simulink model "TP3_simu_realim_obs_continuo"  (R2023b)
settings: Solver=VariableStepAuto  StartTime=0.0  StopTime=6  FixedStep=20e-3  RelTol=1e-3
values from neighbouring files (symbols this model uses):
  A = sysc .A    [Prueba_Control.m]
  B = sysc .B    [Prueba_Control.m]
  C = sysc .C    [Prueba_Control.m]
  D = sysc .D    [Prueba_Control.m]
  x1e = 0    [Prueba_Control_CI.m]    (also in control3.m)
  x2e = 0    [Prueba_Control_CI.m]    (also in control3.m)
  x3e = 0    [Prueba_Control_CI.m]    (also in control3.m)
  x4e = 0    [Prueba_Control_CI.m]    (also in control3.m)
undefined symbols (not defined in the file or in its folder): Ko, Lo
libraries: cstblocks x1
settings Model: Creator=manuh  LastModifiedBy=ApoloXVIII

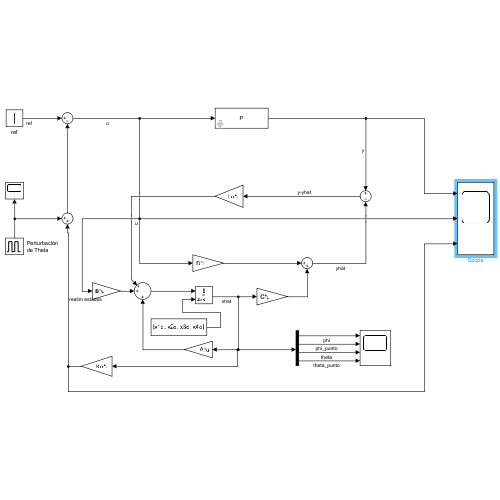
[thumbnail: Simulink's stored preview of the top-level diagram]
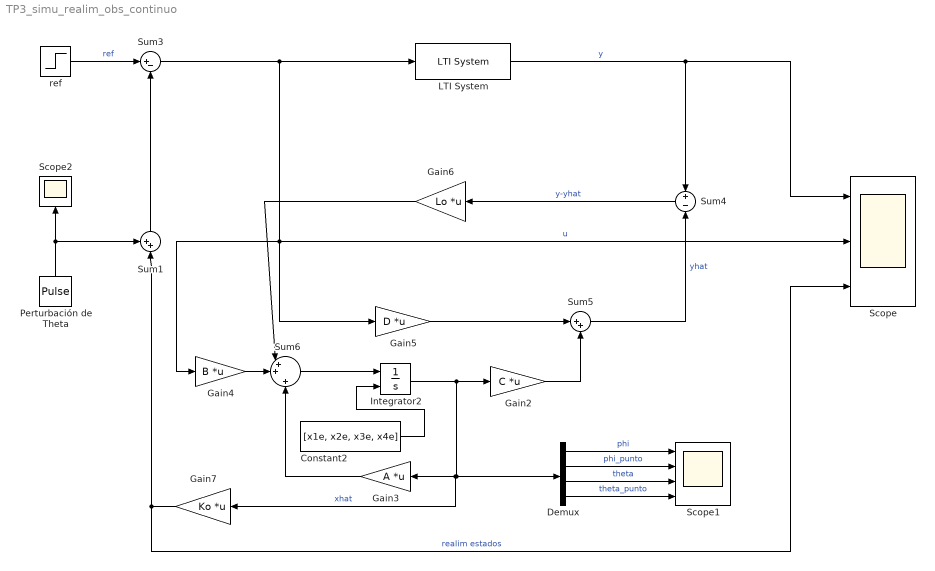
== system TP3_simu_realim_obs_continuo ==
  Constant2 : Constant  Value=[x1e, x2e, x3e, x4e]
  Demux : Demux
  Gain2 : Gain  Gain=C  Multiplication=Matrix(K*u)
  Gain3 : Gain  Gain=A  Multiplication=Matrix(K*u)
  Gain4 : Gain  Gain=B  Multiplication=Matrix(K*u)
  Gain5 : Gain  Gain=D  Multiplication=Matrix(K*u)
  Gain6 : Gain  Gain=Lo  Multiplication=Matrix(K*u)
  Gain7 : Gain  Gain=Ko  Multiplication=Matrix(K*u)
  Integrator2 : Integrator  InitialConditionSource=external
  LTI System : cstblocks/LTI System  sys=P  IC=[]  PadeOrder=0
  Perturbación de Theta : DiscretePulseGenerator  PulseType=Time based  Amplitude=-30  Period=12  PulseWidth=0.1  PhaseDelay=2
  Scope : Scope  NumInputPorts=3
  Scope1 : Scope  NumInputPorts=4
  Scope2 : Scope
  Sum1 : Sum  Inputs=++|
  Sum3 : Sum  Inputs=|+-
  Sum4 : Sum  Inputs=+|-
  Sum5 : Sum  Inputs=|++
  Sum6 : Sum  Inputs=|++|+
  ref : Step  Time=0  After=0  SampleTime=0
  wires:
  ref/1 -> Sum3/1  "ref"
  Sum3/1 -> Scope/2, Gain5/1, Gain4/1, LTI System/1  "u"
  Sum4/1 -> Gain6/1  "y-yhat"
  LTI System/1 -> Sum4/1, Scope/1  "y"
  Gain5/1 -> Sum5/1
  Sum5/1 -> Sum4/2  "yhat"
  Gain2/1 -> Sum5/2
  Integrator2/1 -> Gain7/1, Gain3/1, Demux/1, Gain2/1  "xhat"
  Gain3/1 -> Sum6/3
  Sum6/1 -> Integrator2/1
  Gain4/1 -> Sum6/2
  Gain6/1 -> Sum6/1
  Constant2/1 -> Integrator2/2
  Gain7/1 -> Sum1/2, Scope/3  "realim estados"
  Demux/1 -> Scope1/1  "phi"
  Demux/2 -> Scope1/2  "phi_punto"
  Demux/3 -> Scope1/3  "theta"
  Demux/4 -> Scope1/4  "theta_punto"
  Perturbación de Theta/1 -> Sum1/1, Scope2/1
  Sum1/1 -> Sum3/2
